simulink model "HILArduinoBici"  (R2015a)
settings: Solver=ode3  SolverMode=SingleTasking  StartTime=0.0  StopTime=6  FixedStep=0.001  RelTol=1e-3
libraries: instrumentlib x2
settings Model: Creator=cinvestavguadalajara  LastModifiedBy=edwar
settings DataIOCC: SignalLoggingSaveFormat=ModelDataLogs
settings DebuggingCC: SolverPrmCheckMsg=warning  MultiTaskDSMMsg=warning  MultiTaskCondExecSysMsg=none  BusObjectLabelMismatch=error  RootOutportRequireBusObject=error

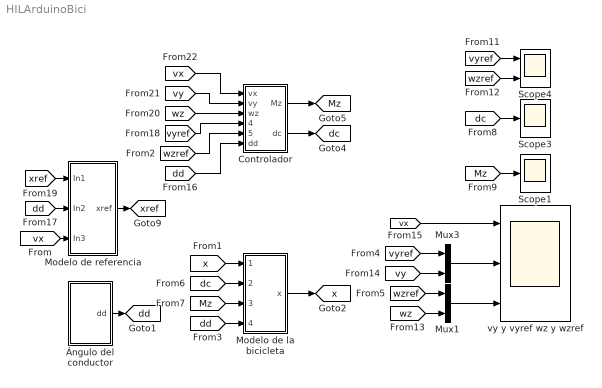
== system HILArduinoBici ==
  Controlador : Subsystem
  Modelo de la bicicleta : Subsystem
  Modelo de referencia : Subsystem
  Mux1 : Mux  Inputs=2
  Mux3 : Mux  Inputs=2
  Scope1 : Scope
      settings: TimeRange=10  YMin=-0.2  YMax=0.15  SaveName=dd1  DataFormat=Structure
  Scope3 : Scope
      settings: TimeRange=10  YMin=0.412545  YMax=0.412635  SaveName=dd  DataFormat=Structure
  Scope4 : Scope  NumInputPorts=2
      settings: TimeRange=10  YMin=-1.5~-0.8  YMax=2~0.6000000000000001  SaveName=dd3  DataFormat=Structure
  "vy y vyref wz y wzref " : Scope  NumInputPorts=3
      settings: TimeRange=6  YMin=27.5~-2.5~0  YMax=28.1~0.5~0.6000000000000001
  "Ángulo del conductor " : Subsystem
  tag scope: Mz=global, dc=global, dd=global, x=global, xref=global
  wires:
  [vyref] -> Mux3/1
  Mux3/1 -> "vy y vyref wz y wzref "/2
  Mux1/1 -> "vy y vyref wz y wzref "/3
  [dc] -> Scope3/1
  [Mz] -> Scope1/1
  [vyref] -> Scope4/1
  [wzref] -> Scope4/2
  [wz] -> Mux1/2
  [vy] -> Mux3/2
  [vx] -> "vy y vyref wz y wzref "/1
  Modelo de referencia/1(xref) -> [xref]
  "Ángulo del conductor "/1(dd) -> [dd]
  [x] -> Modelo de la bicicleta/1(1)
  [dc] -> Modelo de la bicicleta/2(2)
  [Mz] -> Modelo de la bicicleta/3(3)
  [dd] -> Modelo de la bicicleta/4(4)
  Modelo de la bicicleta/1(x) -> [x]
  [xref] -> Modelo de referencia/1(In1)
  [dd] -> Modelo de referencia/2(In2)
  [vx] -> Modelo de referencia/3(In3)
  [wzref] -> Mux1/1
  [vx] -> Controlador/1(vx)
  [vy] -> Controlador/2(vy)
  [wz] -> Controlador/3(wz)
  [dd] -> Controlador/6(dd)
  [vyref] -> Controlador/4(vyref)
  [wzref] -> Controlador/5(wzref)
  Controlador/2(dc) -> [dc]
  Controlador/1(Mz) -> [Mz]

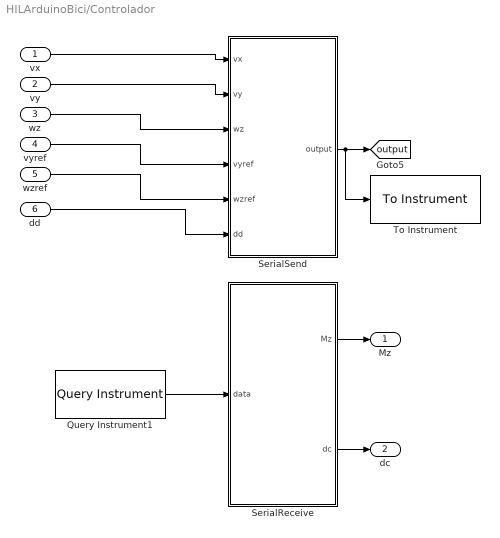
== system HILArduinoBici/Controlador ==
  vx : Inport
  vy : Inport  Port=2
  wz : Inport  Port=3
  vyref : Inport  Port=4
  wzref : Inport  Port=5
  dd : Inport  Port=6
  Query Instrument1 : instrumentlib/Query Instrument  Priority=2  sampleTime=inf  isWorkspaceObject=on  timeout=10  inputBufferSize=512  protocol=Serial  serialPort=COM1  baudRate=9600  gpibVendor=Advantech  boardIndex=0  primaryAddress=1  secondaryAddress=0  visaVendor=Agilent  visaSerialPort=0  chassisIndex=0  logicalAddress=0  tcpRemoteHost='127.0.0.1'  tcpRemotePort=4500  udpRemoteHost='127.0.0.1'  udpRemotePort=9090  visaTCPBoardIndex=0  visaTCPRemoteHost='127.0.0.1'  usbBoardIndex=0  usbManufID=0  usbModelCode=0  usbSerialNumber=0  wsVariableName=port  initAction=Send ASCII Commands  initCommand=''  initFunction=get  queryCommand=''  responseFormat=ASCII  asciiFormatting='%f,%f'  precision=8-bit integer  byteOrder=Little Endian  valuesToRead=1  removeBytes=on  afterOutputAction=Repeat query for new data  enableFrames=on  frameSize=2
  "SerialReceive " : MATLAB Function  TreatAsAtomicUnit=on
  SerialSend : MATLAB Function  TreatAsAtomicUnit=on
  To Instrument : instrumentlib/To Instrument  Priority=1  sampleTime=-1  isWorkspaceObject=on  timeout=10  inputBufferSize=8192  protocol=Serial  serialPort=COM1  baudRate=9600  gpibVendor=Advantech  boardIndex=0  primaryAddress=1  secondaryAddress=0  visaVendor=Agilent  visaSerialPort=0  chassisIndex=0  logicalAddress=0  tcpRemoteHost='127.0.0.1'  tcpRemotePort=4500  udpRemoteHost='127.0.0.1'  udpRemotePort=9090  visaTCPBoardIndex=0  visaTCPRemoteHost='127.0.0.1'  usbBoardIndex=0  usbManufID=0  usbModelCode=0  usbSerialNumber=0  wsVariableName=port  initAction=Send ASCII Commands  initCommand='|start'  initFunction=get  command=''  sendFormat=ASCII  asciiFormatting='|%04.4e,%04.4e,%04.4e,%04.4e,%04.4e,%04.4e\n'  precision=8-bit integer  byteOrder=Little Endian
  Mz : Outport
  dc : Outport  Port=2
  tag scope: output=global
  wires:
  SerialSend/1(output) -> To Instrument/1, [output]
  vx/1 -> SerialSend/1(vx)
  vy/1 -> SerialSend/2(vy)
  wz/1 -> SerialSend/3(wz)
  vyref/1 -> SerialSend/4(vyref)
  wzref/1 -> SerialSend/5(wzref)
  dd/1 -> SerialSend/6(dd)
  "SerialReceive "/1(Mz) -> Mz/1
  "SerialReceive "/2(dc) -> dc/1
  Query Instrument1/1 -> "SerialReceive "/1(data)

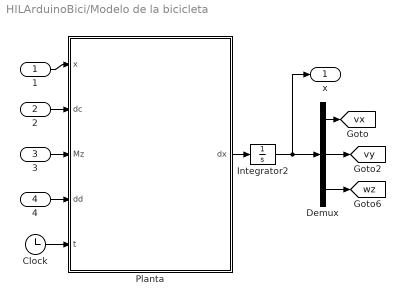
== system HILArduinoBici/Modelo de la bicicleta ==
  1 : Inport
  2 : Inport  Port=2
  3 : Inport  Port=3
  4 : Inport  Port=4
  Clock : Clock
  Demux : Demux  Outputs=3
  Integrator2 : Integrator  InitialCondition=[28 0 0]
  Planta : MATLAB Function  TreatAsAtomicUnit=on
  x : Outport
  tag scope: vx=global, vy=global, wz=global
  wires:
  Demux/3 -> [wz]
  Demux/2 -> [vy]
  Demux/1 -> [vx]
  Planta/1(dx) -> Integrator2/1
  Integrator2/1 -> x/1, Demux/1
  1/1 -> Planta/1(x)
  2/1 -> Planta/2(dc)
  3/1 -> Planta/3(Mz)
  4/1 -> Planta/4(dd)
  Clock/1 -> Planta/5(t)

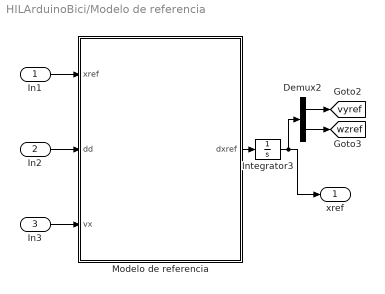
== system HILArduinoBici/Modelo de referencia ==
  In1 : Inport
  In2 : Inport  Port=2
  In3 : Inport  Port=3
  Demux2 : Demux  Outputs=2
  Integrator3 : Integrator  InitialCondition=[0 0]
  Modelo de referencia : MATLAB Function  TreatAsAtomicUnit=on
  xref : Outport
  tag scope: vyref=global, wzref=global
  wires:
  Integrator3/1 -> xref/1, Demux2/1
  Demux2/1 -> [vyref]
  Demux2/2 -> [wzref]
  Modelo de referencia/1(dxref) -> Integrator3/1
  In1/1 -> Modelo de referencia/1(xref)
  In2/1 -> Modelo de referencia/2(dd)
  In3/1 -> Modelo de referencia/3(vx)

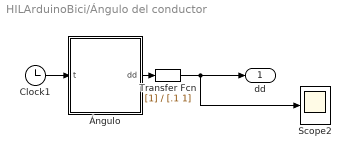
== system HILArduinoBici/Ángulo del conductor  ==
  Clock1 : Clock
  Scope2 : Scope
      settings: TimeRange=10  YMin=-0.2  YMax=0.15  SaveName=dd2  DataFormat=Structure
  Transfer Fcn : TransferFcn  Denominator=[.1 1]
  Ángulo : MATLAB Function  TreatAsAtomicUnit=on
  dd : Outport
  wires:
  Ángulo/1(dd) -> Transfer Fcn/1
  Clock1/1 -> Ángulo/1(t)
  Transfer Fcn/1 -> dd/1, Scope2/1

== matlab function HILArduinoBici/Modelo de la bicicleta/Planta ==
  data: x input; dx output; dc input; Mz input; dd input; t input
function dx=fcn(x,dc,Mz,dd,t)
vx=x(1);
vy=x(2);
wz=x(3);
 
Lf = 1.17; 
Lr = 1.43; 
Cf= 1.81;
Cr=1.68;
Bf=7.2;
Br=11;
Dr=8394;
Df=8854;
m = 1480; 
Jz = 2300; 

mu=0.9;
if t<1
    mu=0.9;
elseif t<2.8
    mu=0.5;
% else
%     mu=0.4;
end

alphar=-(vy-Lr*wz)/vx;
phir=sin(Cr*atan(Br*alphar));

alphaf0=dd-(vy+Lf*wz)/vx;
phif0=sin(Cf*atan(Bf*alphaf0));

alphaf=dd+dc-(vy+Lf*wz)/vx;
phif=sin(Cf*atan(Bf*(alphaf)));

Fyr=Dr*phir;
Fyf=Df*phif;

ay=(mu/m)*(Fyf+Fyr);

Dc=phif-phif0;

dvx=vy*wz;
dvy=-vx*wz+(mu/m)*(Df*phif0+Dr*phir)+(mu/m)*Df*Dc;
dwz=(mu/Jz)*(Df*phif0*Lf-Dr*phir*Lr)+(mu/Jz)*Df*Lf*Dc+(1/Jz)*Mz;


dx=[dvx dvy dwz];

== matlab function HILArduinoBici/Ángulo del conductor /Ángulo ==
  data: t input; dd output
function dd = fcn(t)

% if t<1
%     dd=0;
% elseif t<2
%       dd=(100*pi/(16*180));
% elseif t<3
%       dd=-(100*pi/(16*180));
% else
%      dd=0;
% end

if t<0.5
    dd=0;
elseif t<2.5
      dd=(359*pi/(16*180));
elseif t<3.5
      dd=-(359*pi/(16*180));
else
     dd=0;
end

== matlab function HILArduinoBici/Controlador/SerialSend ==
  data: vx input; vy input; wz input; vyref input; wzref input; output output; dd input
function output = fcn(vx, vy, wz, vyref, wzref, dd)

output = [vx, vy, wz, vyref, wzref, dd];

== matlab function HILArduinoBici/Modelo de referencia/Modelo de referencia ==
  data: xref input; dd input; vx input; dxref output
function dxref=fcn(xref,dd,vx)

vyref=xref(1);
wzref=xref(2);

Lf = 1.17; 
Lr = 1.43; 
Cf= 1.81;
Cr=1.68;
Bf=7.2;
Br=11;
Dr=8394;
Df=8854;
m = 1480; 
Jz = 2300; 

mu=.9;

alphaf0_ref=dd-(vyref+Lf*wzref)/vx;
alphar_ref=-(vyref-Lr*wzref)/vx;

phif0ref=sin(Cf*atan(Bf*(alphaf0_ref)));
phirref=sin(Cr*atan(Br*(alphar_ref)));

dvyref=-vx*wzref+(mu/m)*(Df*phif0ref+Dr*phirref);
dwzref=(mu/Jz)*(Df*phif0ref*Lf-Dr*phirref*Lr);

dxref= [dvyref dwzref];

== matlab function HILArduinoBici/Controlador/SerialReceive  ==
  data: Mz output; dc output; data input
function [Mz, dc] = fcn(data)


%Mz = 1;
%dc = 2;
Mz = data(1);
dc = data(2);
